simulink model "fuzzy_pid_control_kp_part"  (R2016a)
settings: Solver=VariableStepAuto  StartTime=0.0  StopTime=10.0  RelTol=1e-3
settings Model: SnapshotBufferSize=1  Creator=Shinelon  LastModifiedBy=Shinelon

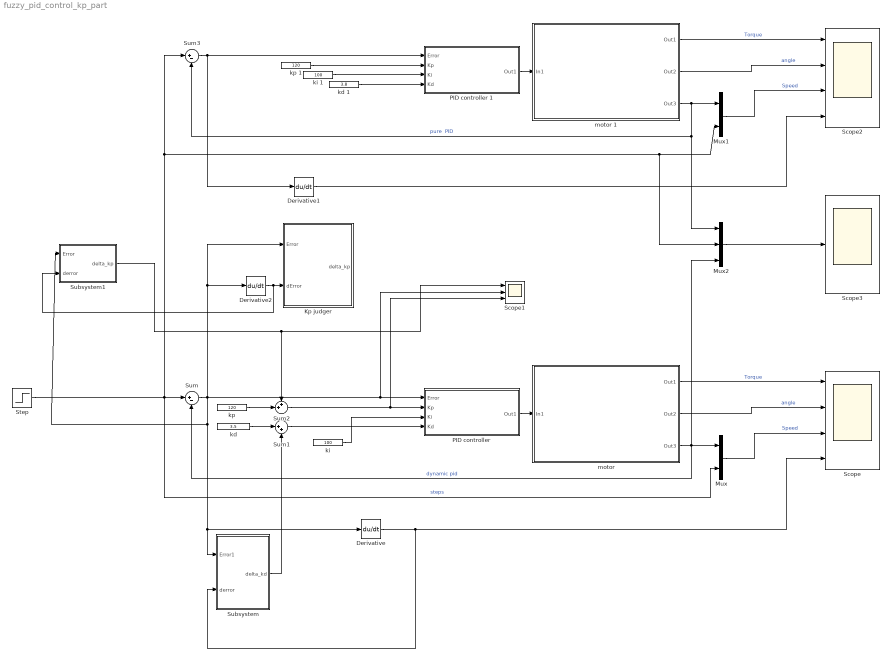
== system fuzzy_pid_control_kp_part ==
  Derivative : Derivative
  Derivative1 : Derivative
  Derivative2 : Derivative
  "Kp judger " : Subsystem
  Mux : Mux  Inputs=2
  Mux1 : Mux  Inputs=2
  Mux2 : Mux  Inputs=3
  "PID controller " : Subsystem
  PID controller 1 : Subsystem
  Scope : Scope  NumInputPorts=4
  Scope1 : Scope  NumInputPorts=3
  Scope2 : Scope  NumInputPorts=4
  Scope3 : Scope
  Step : Step  Time=3  After=20000  SampleTime=0
  Subsystem : Subsystem
  Subsystem1 : Subsystem
  Sum : Sum  Inputs=|+-
  Sum1 : Sum  Inputs=|++
  Sum2 : Sum  Inputs=++|
  Sum3 : Sum  Inputs=|+-
  "kd " : Constant  Value=3.5
  kd 1 : Constant  Value=3.8
  "ki " : Constant  Value=100
  ki 1 : Constant  Value=100
  "kp " : Constant  Value=120
  kp 1 : Constant  Value=120
  "motor " : Subsystem  mask(DC motor subsystem){R=2, L=0.5, Km=0.1, Kf=0.2, Kemf=0.1, J=0.02}
      mask prompts: R "Resistor"; L "Inductor"; Km "Torque Constant"; Kf "Viscous Friction Constant"; Kemf "Back EMF Votage Constant"; J "Inertial Load"
      mask help:
      | This is a DC motor subsystem
      | Input : Control Signal
      | Output : Motor Rate
      mask init:
      | R=2;
      | L=0.5;
      | Km=0.1;
      | Kemf=0.1;
      | Kf=0.2;
      | J=0.02;
      mask Display:
      | color('red');port_label('input',1,'Control Signal');
      | color('red');port_label('output',1,'Torque');
      | color('red');port_label('output',2,'Angle');
      | color('red');port_label('output',3,'Speed');
      | image(imread('E:\simulink model\DC motor model\timg.jpg'))
  motor 1 : Subsystem  mask(DC motor subsystem){R=2, L=0.5, Km=0.1, Kf=0.2, Kemf=0.1, J=0.02}
      mask prompts: R "Resistor"; L "Inductor"; Km "Torque Constant"; Kf "Viscous Friction Constant"; Kemf "Back EMF Votage Constant"; J "Inertial Load"
      mask help:
      | This is a DC motor subsystem
      | Input : Control Signal
      | Output : Motor Rate
      mask init:
      | R=2;
      | L=0.5;
      | Km=0.1;
      | Kemf=0.1;
      | Kf=0.2;
      | J=0.02;
      mask Display:
      | color('red');port_label('input',1,'Control Signal');
      | color('red');port_label('output',1,'Torque');
      | color('red');port_label('output',2,'Angle');
      | color('red');port_label('output',3,'Speed');
      | image(imread('E:\simulink model\DC motor model\timg.jpg'))
  wires:
  "motor "/1(Out1) -> Scope/1  "Torque"
  "motor "/2(Out2) -> Scope/2  "angle"
  "motor "/3(Out3) -> Mux2/3, Sum/2, Mux/1  "dynamic pid"
  "PID controller "/1(Out1) -> "motor "/1(In1)
  Derivative/1 -> Subsystem/2(derror), Scope/4
  Mux/1 -> Scope/3  "Speed"
  Sum/1 -> Subsystem1/1(Error), Subsystem/1(Error1), Derivative/1, Derivative2/1, "Kp judger "/1(Error), Scope1/2, "PID controller "/1("Error ")
  "ki "/1 -> "PID controller "/3("Ki ")
  "kp "/1 -> Sum2/2
  Sum2/1 -> Scope1/3, "PID controller "/2("Kp ")
  motor 1/1(Out1) -> Scope2/1  "Torque"
  motor 1/2(Out2) -> Scope2/2  "angle"
  motor 1/3(Out3) -> Mux2/1, Sum3/2, Mux1/1  "pure  PID"
  Step/1 -> Sum3/1, Mux2/2, Mux1/2, Mux/2, Sum/1  "steps"
  PID controller 1/1(Out1) -> motor 1/1(In1)
  Derivative1/1 -> Scope2/4
  Mux1/1 -> Scope2/3  "Speed"
  Sum3/1 -> PID controller 1/1("Error "), Derivative1/1
  ki 1/1 -> PID controller 1/3("Ki ")
  kd 1/1 -> PID controller 1/4(Kd)
  kp 1/1 -> PID controller 1/2("Kp ")
  Mux2/1 -> Scope3/1
  Derivative2/1 -> Subsystem1/2(derror), "Kp judger "/2(dError)
  "kd "/1 -> Sum1/1
  Sum1/1 -> "PID controller "/4(Kd)
  Subsystem1/1("delta_kp ") -> Scope1/1, Sum2/1
  Subsystem/1("delta_kd ") -> Sum1/2

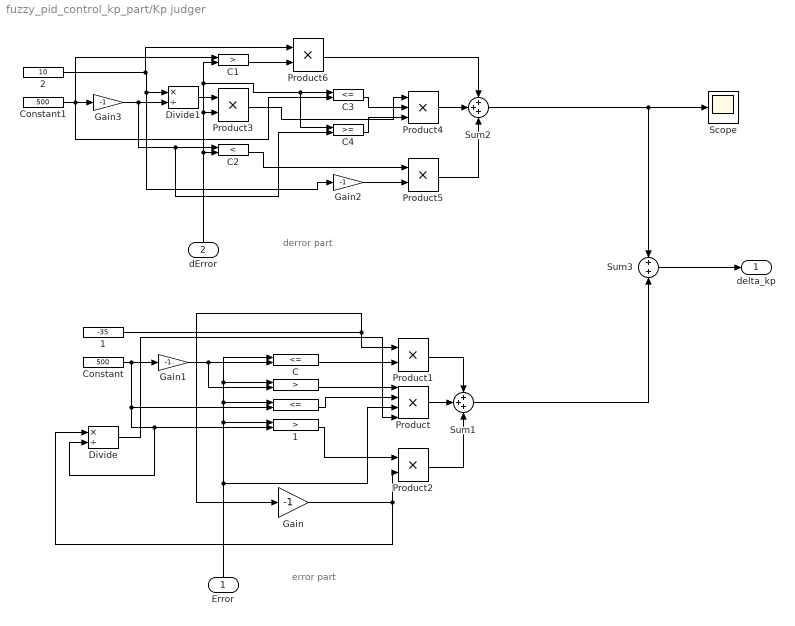
== system fuzzy_pid_control_kp_part/Kp judger  ==
  note: error part
  note: derror part
  Error : Inport
  dError : Inport  Port=2
  " " : RelationalOperator  Operator=<=  OutDataTypeStr=boolean
  " " : RelationalOperator  Operator=>  OutDataTypeStr=boolean
  " 1" : RelationalOperator  Operator=>  OutDataTypeStr=boolean
  "1 " : Constant  Value=-35
  "2 " : Constant  Value=10
  "C " : RelationalOperator  Operator=<=  OutDataTypeStr=boolean
  C1 : RelationalOperator  Operator=>  OutDataTypeStr=boolean
  C2 : RelationalOperator  Operator=<  OutDataTypeStr=boolean
  C3 : RelationalOperator  Operator=<=  OutDataTypeStr=boolean
  C4 : RelationalOperator  OutDataTypeStr=boolean
  Constant : Constant  Value=500
  Constant1 : Constant  Value=500
  Divide : Product  Inputs=*/
  Divide1 : Product  Inputs=*/
  Gain{,1..3} (4 alike) : Gain  Gain=-1
  Product : Product  Inputs=4
  Product{1..3,5..6} (5 alike) : Product
  Product4 : Product  Inputs=3
  Scope : Scope
  Sum1 : Sum  Inputs=+++
  Sum2 : Sum  Inputs=+++
  Sum3 : Sum  Inputs=+|+
  "delta_kp " : Outport
  wires:
  Product/1 -> Sum1/2
  Product2/1 -> Sum1/3
  " "/1 -> Product/2
  " "/1 -> Product/1
  " 1"/1 -> Product2/1
  Constant/1 -> " "/2, Divide/2, " 1"/2, Gain1/1
  Divide/1 -> Product/4
  "C "/1 -> Product1/2
  Gain/1 -> Divide/1, Product2/2
  "1 "/1 -> Gain/1, Product1/1
  Error/1 -> Product/3, " 1"/1, " "/1, " "/1, "C "/1
  Gain1/1 -> " "/2, "C "/2
  Product1/1 -> Sum1/1
  Constant1/1 -> C1/1, C3/2, Gain3/1
  Sum3/1 -> "delta_kp "/1
  Sum1/1 -> Sum3/2
  Gain3/1 -> C4/2, C2/1, Divide1/2
  "2 "/1 -> Product6/1, Gain2/1, Divide1/1
  Divide1/1 -> Product3/1
  dError/1 -> C2/2, C1/2, C4/1, C3/1, Product3/2
  C1/1 -> Product6/2
  Product6/1 -> Sum2/1
  C2/1 -> Product5/1
  Product4/1 -> Sum2/2
  Product3/1 -> Product4/1
  C4/1 -> Product4/3
  C3/1 -> Product4/2
  Sum2/1 -> Sum3/1, Scope/1
  Gain2/1 -> Product5/2
  Product5/1 -> Sum2/3

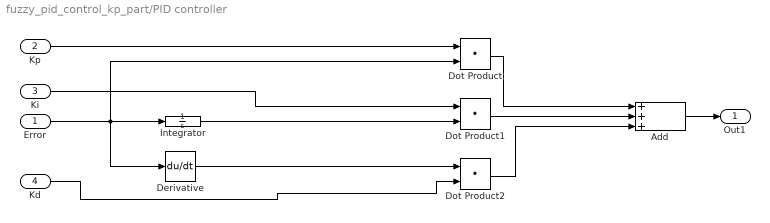
== system fuzzy_pid_control_kp_part/PID controller  ==
  "Error " : Inport
  "Kp " : Inport  Port=2
  "Ki " : Inport  Port=3
  Kd : Inport  Port=4
  Add : Sum  Inputs=+++
  Derivative : Derivative
  Dot Product : DotProduct  InputSameDT=on  OutDataTypeStr=Inherit: Inherit via internal rule
  Dot Product1 : DotProduct  InputSameDT=on  OutDataTypeStr=Inherit: Inherit via internal rule
  Dot Product2 : DotProduct  InputSameDT=on  OutDataTypeStr=Inherit: Inherit via internal rule
  Integrator : Integrator
  Out1 : Outport
  wires:
  Integrator/1 -> Dot Product1/2
  Dot Product2/1 -> Add/3
  "Error "/1 -> Dot Product/2, Integrator/1, Derivative/1
  Derivative/1 -> Dot Product2/1
  Dot Product/1 -> Add/1
  "Ki "/1 -> Dot Product1/1
  Add/1 -> Out1/1
  Kd/1 -> Dot Product2/2
  Dot Product1/1 -> Add/2
  "Kp "/1 -> Dot Product/1

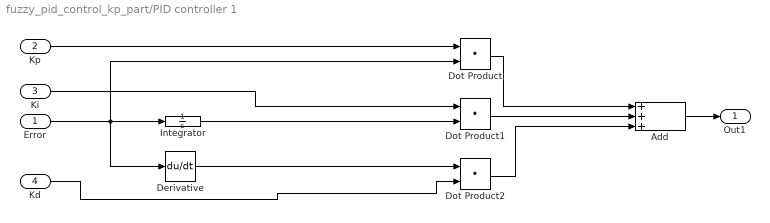
== system fuzzy_pid_control_kp_part/PID controller 1 ==
  "Error " : Inport
  "Kp " : Inport  Port=2
  "Ki " : Inport  Port=3
  Kd : Inport  Port=4
  Add : Sum  Inputs=+++
  Derivative : Derivative
  Dot Product : DotProduct  InputSameDT=on  OutDataTypeStr=Inherit: Inherit via internal rule
  Dot Product1 : DotProduct  InputSameDT=on  OutDataTypeStr=Inherit: Inherit via internal rule
  Dot Product2 : DotProduct  InputSameDT=on  OutDataTypeStr=Inherit: Inherit via internal rule
  Integrator : Integrator
  Out1 : Outport
  wires:
  Integrator/1 -> Dot Product1/2
  Dot Product2/1 -> Add/3
  "Error "/1 -> Dot Product/2, Integrator/1, Derivative/1
  Derivative/1 -> Dot Product2/1
  Dot Product/1 -> Add/1
  "Ki "/1 -> Dot Product1/1
  Add/1 -> Out1/1
  Kd/1 -> Dot Product2/2
  Dot Product1/1 -> Add/2
  "Kp "/1 -> Dot Product/1

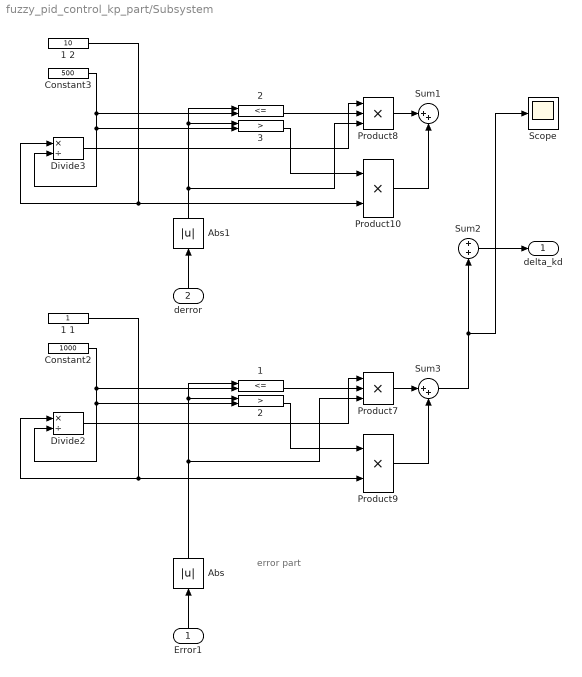
== system fuzzy_pid_control_kp_part/Subsystem ==
  note: error part
  Error1 : Inport
  derror : Inport  Port=2
  " 2" : RelationalOperator  Operator=>  OutDataTypeStr=boolean
  " 3" : RelationalOperator  Operator=>  OutDataTypeStr=boolean
  " 1" : RelationalOperator  Operator=<=  OutDataTypeStr=boolean
  " 2" : RelationalOperator  Operator=<=  OutDataTypeStr=boolean
  1 1 : Constant
  1 2 : Constant  Value=10
  Abs : Abs
  Abs1 : Abs
  Constant2 : Constant  Value=1000
  Constant3 : Constant  Value=500
  Divide2 : Product  Inputs=*/
  Divide3 : Product  Inputs=*/
  Product10 : Product
  Product7 : Product  Inputs=3
  Product8 : Product  Inputs=3
  Product9 : Product
  Scope : Scope
  Sum1 : Sum  Inputs=|++
  Sum2 : Sum  Inputs=+|+
  Sum3 : Sum  Inputs=|++
  "delta_kd " : Outport
  wires:
  Divide2/1 -> Product7/1
  Constant2/1 -> Divide2/2, " 2"/2, " 1"/2
  " 1"/1 -> Product7/2
  1 1/1 -> Divide2/1, Product9/2
  " 2"/1 -> Product9/1
  Product7/1 -> Sum3/1
  Product9/1 -> Sum3/2
  Error1/1 -> Abs/1
  Abs/1 -> Product7/3, " 1"/1, " 2"/1
  Divide3/1 -> Product8/1
  Constant3/1 -> Divide3/2, " 3"/2, " 2"/2
  " 2"/1 -> Product8/2
  1 2/1 -> Divide3/1, Product10/2
  " 3"/1 -> Product10/1
  Product8/1 -> Sum1/1
  Product10/1 -> Sum1/2
  Sum2/1 -> "delta_kd "/1
  Sum3/1 -> Scope/1, Sum2/2
  Abs1/1 -> Product8/3, " 2"/1, " 3"/1
  derror/1 -> Abs1/1

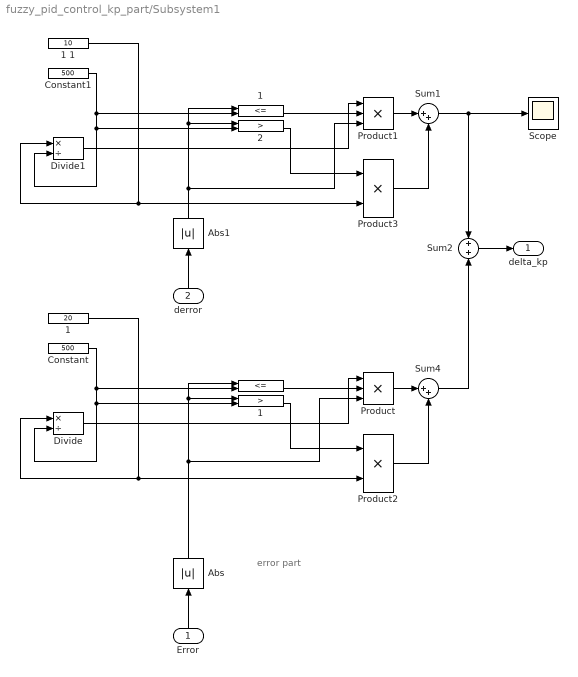
== system fuzzy_pid_control_kp_part/Subsystem1 ==
  note: error part
  Error : Inport
  derror : Inport  Port=2
  " " : RelationalOperator  Operator=<=  OutDataTypeStr=boolean
  " 1" : RelationalOperator  Operator=>  OutDataTypeStr=boolean
  " 2" : RelationalOperator  Operator=>  OutDataTypeStr=boolean
  " 1" : RelationalOperator  Operator=<=  OutDataTypeStr=boolean
  "1 " : Constant  Value=20
  1 1 : Constant  Value=10
  Abs : Abs
  Abs1 : Abs
  Constant : Constant  Value=500
  Constant1 : Constant  Value=500
  Divide : Product  Inputs=*/
  Divide1 : Product  Inputs=*/
  Product : Product  Inputs=3
  Product1 : Product  Inputs=3
  Product2 : Product
  Product3 : Product
  Scope : Scope
  Sum1 : Sum  Inputs=|++
  Sum2 : Sum  Inputs=+|+
  Sum4 : Sum  Inputs=|++
  "delta_kp " : Outport
  wires:
  Divide/1 -> Product/1
  Constant/1 -> Divide/2, " 1"/2, " "/2
  " "/1 -> Product/2
  "1 "/1 -> Divide/1, Product2/2
  " 1"/1 -> Product2/1
  Product/1 -> Sum4/1
  Product2/1 -> Sum4/2
  Error/1 -> Abs/1
  Abs/1 -> Product/3, " "/1, " 1"/1
  Divide1/1 -> Product1/1
  Constant1/1 -> Divide1/2, " 2"/2, " 1"/2
  " 1"/1 -> Product1/2
  1 1/1 -> Divide1/1, Product3/2
  " 2"/1 -> Product3/1
  Product1/1 -> Sum1/1
  Product3/1 -> Sum1/2
  Sum2/1 -> "delta_kp "/1
  Sum1/1 -> Scope/1, Sum2/1
  Sum4/1 -> Sum2/2
  Abs1/1 -> Product1/3, " 1"/1, " 2"/1
  derror/1 -> Abs1/1

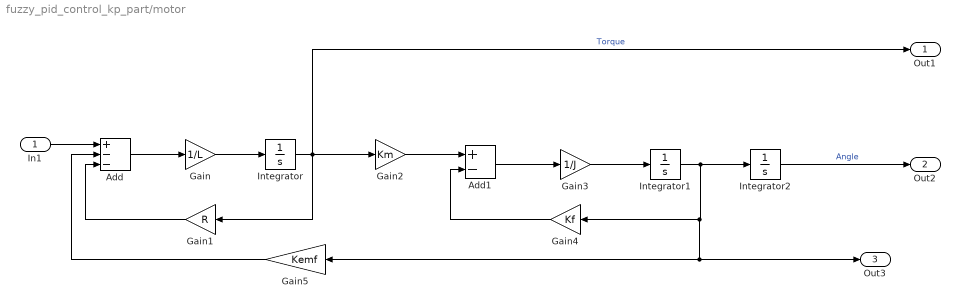
== system fuzzy_pid_control_kp_part/motor  ==
  In1 : Inport
  Add : Sum  Inputs=+--
  Add1 : Sum  Inputs=+-
  Gain : Gain  Gain=1/L
  Gain1 : Gain  Gain=R
  Gain2 : Gain  Gain=Km
  Gain3 : Gain  Gain=1/J
  Gain4 : Gain  Gain=Kf
  Gain5 : Gain  Gain=Kemf
  Integrator : Integrator
  Integrator1 : Integrator
  Integrator2 : Integrator
  Out1 : Outport
  Out2 : Outport  Port=2
  Out3 : Outport  Port=3
  wires:
  Gain5/1 -> Add/2
  Integrator/1 -> Out1/1, Gain2/1, Gain1/1  "Torque"
  Integrator2/1 -> Out2/1  "Angle"
  Add/1 -> Gain/1
  Gain/1 -> Integrator/1
  Gain1/1 -> Add/3
  Gain2/1 -> Add1/1
  Add1/1 -> Gain3/1
  Gain3/1 -> Integrator1/1
  Integrator1/1 -> Integrator2/1, Out3/1, Gain5/1, Gain4/1
  Gain4/1 -> Add1/2
  In1/1 -> Add/1

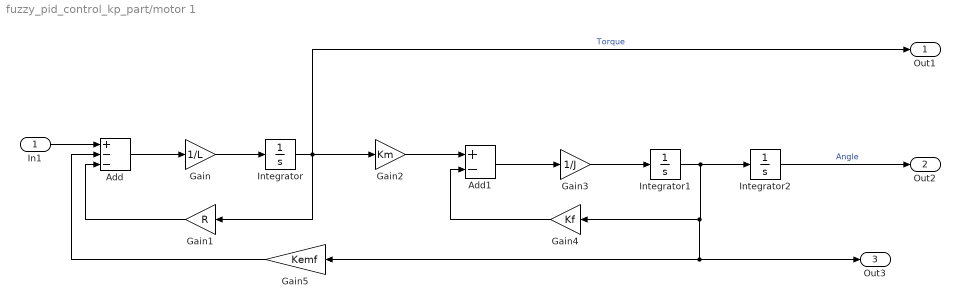
== system fuzzy_pid_control_kp_part/motor 1 ==
  In1 : Inport
  Add : Sum  Inputs=+--
  Add1 : Sum  Inputs=+-
  Gain : Gain  Gain=1/L
  Gain1 : Gain  Gain=R
  Gain2 : Gain  Gain=Km
  Gain3 : Gain  Gain=1/J
  Gain4 : Gain  Gain=Kf
  Gain5 : Gain  Gain=Kemf
  Integrator : Integrator
  Integrator1 : Integrator
  Integrator2 : Integrator
  Out1 : Outport
  Out2 : Outport  Port=2
  Out3 : Outport  Port=3
  wires:
  Gain5/1 -> Add/2
  Integrator/1 -> Out1/1, Gain2/1, Gain1/1  "Torque"
  Integrator2/1 -> Out2/1  "Angle"
  Add/1 -> Gain/1
  Gain/1 -> Integrator/1
  Gain1/1 -> Add/3
  Gain2/1 -> Add1/1
  Add1/1 -> Gain3/1
  Gain3/1 -> Integrator1/1
  Integrator1/1 -> Integrator2/1, Out3/1, Gain5/1, Gain4/1
  Gain4/1 -> Add1/2
  In1/1 -> Add/1
